simulink model "dataget_simu"  (R2024a)
settings: Solver=FixedStepDiscrete  StartTime=0.0  StopTime=time  FixedStep=ts  RelTol=1e-3
undefined symbols (not defined in the file): A, A0, A_aspr, B, B0, B_aspr, C, C0, C_aspr, D, D0, D_aspr, sam_time, seed, ts
libraries: simulink x1
settings Model: Creator=lenovo  LastModifiedBy=lenovo

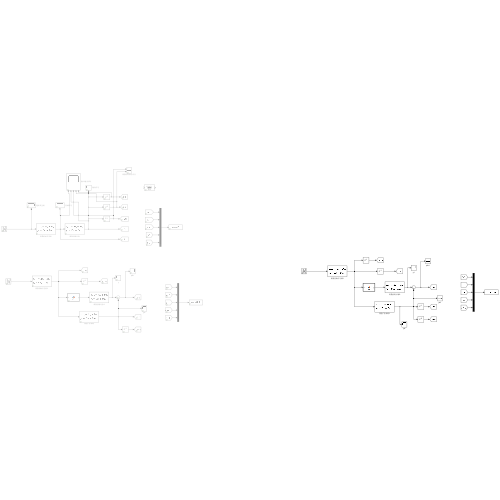
[thumbnail: Simulink's stored preview of the top-level diagram]
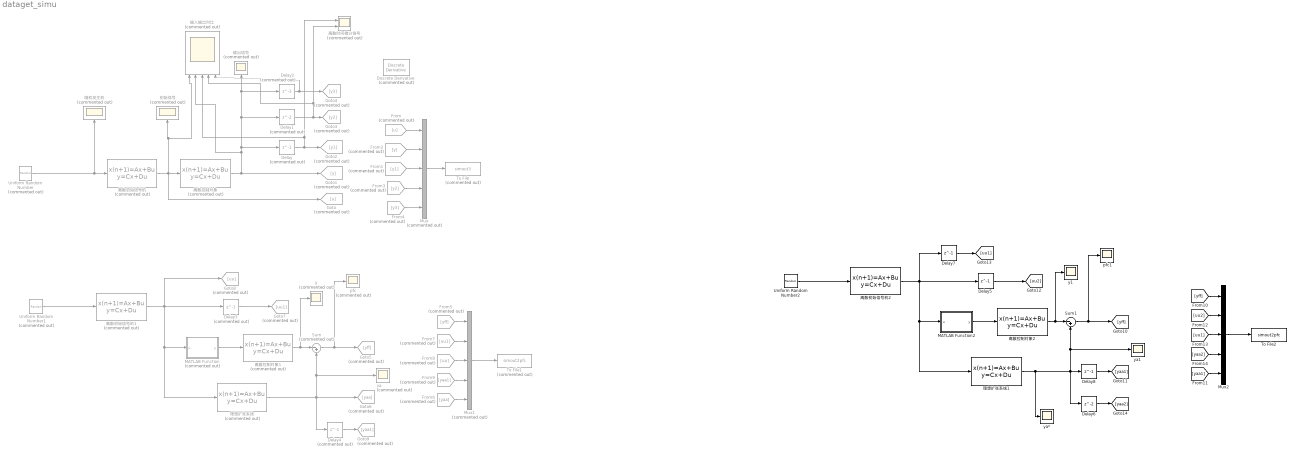
== system dataget_simu ==
  Delay : Delay  Commented=on  DelayLength=1  InitialCondition=0
  Delay1 : Delay  Commented=on  InitialCondition=0
  Delay2 : Delay  Commented=on  DelayLength=3  InitialCondition=0
  Delay3 : Delay  Commented=on  DelayLength=1  InitialCondition=0
  Delay4 : Delay  Commented=on  DelayLength=1  InitialCondition=0
  Delay5 : Delay  DelayLength=1  InitialCondition=0
  Delay6 : Delay  InitialCondition=0
  Delay7 : Delay  DelayLength=1  InitialCondition=0
  Delay8 : Delay  DelayLength=1  InitialCondition=0
  Discrete Derivative : simulink/Discrete/Discrete Derivative  Commented=on  gainval=1.0  ICPrevScaledInput=0.0  OutMin=[]  OutMax=[]  OutDataType=fixdt(1, 16)  OutScaling=2^-10  DoSatur=off
  From : From  Commented=on  GotoTag=u
  From1 : From  Commented=on  GotoTag=y1
  From2 : From  Commented=on  GotoTag=y
  From3 : From  Commented=on  GotoTag=y2
  From4 : From  Commented=on  GotoTag=y3
  From5 : From  Commented=on  GotoTag=yff
  From6 : From  Commented=on  GotoTag=yaa
  From7 : From  Commented=on  GotoTag=uu1
  From8 : From  Commented=on  GotoTag=uu
  From9 : From  Commented=on  GotoTag=yaa1
  Goto : Goto  Commented=on  GotoTag=u
  Goto1 : Goto  Commented=on  GotoTag=y
  Goto2 : Goto  Commented=on  GotoTag=y1
  Goto3 : Goto  Commented=on  GotoTag=y2
  Goto4 : Goto  Commented=on  GotoTag=y3
  Goto5 : Goto  Commented=on  GotoTag=yff
  Goto6 : Goto  Commented=on  GotoTag=yaa
  Goto7 : Goto  Commented=on  GotoTag=uu1
  Goto8 : Goto  Commented=on  GotoTag=uu
  Goto9 : Goto  Commented=on  GotoTag=yaa1
  MATLAB Function : MATLAB Function  Commented=on  TreatAsAtomicUnit=on
  MATLAB Function2 : MATLAB Function  TreatAsAtomicUnit=on
  Mux : Mux  Commented=on  Inputs=5
  Mux1 : Mux  Commented=on  Inputs=5
  Mux2 : Mux  Inputs=5
  Sum : Sum  Commented=on  Inputs=|-+
  Sum1 : Sum  Inputs=|-+
  To File : ToFile  Commented=on  Filename=simout3  MatrixName=simout3  SampleTime=ts
  To File1 : ToFile  Commented=on  Filename=simout2pfc  MatrixName=simout2pfc  SampleTime=ts
  To File2 : ToFile  Filename=simout2pfc  MatrixName=simout2pfc  SampleTime=ts
  Uniform Random Number : UniformRandomNumber  Commented=on  Minimum=0  Maximum=20  Seed=seed  SampleTime=sam_time
  Uniform Random Number1 : UniformRandomNumber  Commented=on  Minimum=0  Maximum=10  Seed=seed  SampleTime=sam_time
  Uniform Random Number2 : UniformRandomNumber  Minimum=0  Maximum=10  Seed=seed  SampleTime=sam_time
  pfc : Scope  Commented=on
  pfc1 : Scope
  y : Scope  Commented=on
  y1 : Scope
  ya : Scope  Commented=on
  ya* : Scope
  ya1 : Scope
  初始信号 : Scope  Commented=on
  理想扩张系统 : DiscreteStateSpace  Commented=on  A=A_aspr  B=B_aspr  C=C_aspr  D=D_aspr  SampleTime=ts
  理想扩张系统1 : DiscreteStateSpace  A=A_aspr  B=B_aspr  C=C_aspr  D=D_aspr  SampleTime=ts
  离散初始信号机 : DiscreteStateSpace  Commented=on  A=A0  B=B0  C=C0  D=D0  SampleTime=ts
  离散初始信号机1 : DiscreteStateSpace  Commented=on  A=A0  B=B0  C=C0  D=D0  SampleTime=ts
  离散初始信号机2 : DiscreteStateSpace  A=A0  B=B0  C=C0  D=D0  SampleTime=ts
  离散控制对象 : DiscreteStateSpace  Commented=on  A=A  B=B  C=C  D=D  SampleTime=ts
  离散控制对象1 : DiscreteStateSpace  Commented=on  A=A  B=B  C=C  D=D  SampleTime=ts
  离散控制对象2 : DiscreteStateSpace  A=A  B=B  C=C  D=D  SampleTime=ts
  离散时间微分信号 : Scope  Commented=on  NumInputPorts=2
  输入输出对比 : Scope  Commented=on  NumInputPorts=5
  输出信号 : Scope  Commented=on
  随机发生机 : Scope  Commented=on
  wires:
  离散控制对象/1 -> Goto1/1, Delay/1, Delay2/1, 输出信号/1, Delay1/1, 输入输出对比/2
  Mux/1 -> To File/1
  离散初始信号机/1 -> 初始信号/1, 输入输出对比/1, 离散控制对象/1, Goto/1
  Delay/1 -> 输入输出对比/3, 离散时间微分信号/1, Goto2/1
  Delay1/1 -> 输入输出对比/4, 离散时间微分信号/2, Goto3/1
  From3/1 -> Mux/4
  From1/1 -> Mux/3
  From2/1 -> Mux/2
  From/1 -> Mux/1
  Delay2/1 -> Goto4/1, 输入输出对比/5
  From4/1 -> Mux/5
  MATLAB Function/1(y) -> 离散控制对象1/1
  Uniform Random Number/1 -> 随机发生机/1, 离散初始信号机/1
  离散控制对象1/1 -> y/1, Sum/1
  理想扩张系统/1 -> Goto6/1, Delay4/1, ya/1, Sum/2
  Sum/1 -> pfc/1, Goto5/1
  Delay3/1 -> Goto7/1
  Uniform Random Number1/1 -> 离散初始信号机1/1
  离散初始信号机1/1 -> Delay3/1, MATLAB Function/1(u), 理想扩张系统/1, Goto8/1
  Delay4/1 -> Goto9/1
  From5/1 -> Mux1/1
  From7/1 -> Mux1/2
  From8/1 -> Mux1/3
  From9/1 -> Mux1/4
  From6/1 -> Mux1/5
  Mux1/1 -> To File1/1
  Sum1/1 -> pfc1/1, [yff]
  Mux2/1 -> To File2/1
  [yff] -> Mux2/1
  Delay5/1 -> [uu2]
  [uu2] -> Mux2/2
  [yaa1] -> Mux2/5
  [uu1] -> Mux2/3
  理想扩张系统1/1 -> ya*/1, Delay8/1, Delay6/1, ya1/1, Sum1/2
  Uniform Random Number2/1 -> 离散初始信号机2/1
  MATLAB Function2/1(y) -> 离散控制对象2/1
  [yaa2] -> Mux2/4
  离散初始信号机2/1 -> Delay5/1, MATLAB Function2/1(u), 理想扩张系统1/1, Delay7/1
  Delay6/1 -> [yaa2]
  离散控制对象2/1 -> y1/1, Sum1/1
  Delay7/1 -> [uu1]
  Delay8/1 -> [yaa1]

== matlab function dataget_simu/MATLAB Function2 ==
  data: u input; y output
function y = fcn(u)

y = 0.06*u^2+0.12*u;

== matlab function dataget_simu/MATLAB Function ==
  data: u input; y output
function y = fcn(u)

y = u^2+2*u;
